simulink subsystem "encoder_8b10b"  (R2022b)
settings: Solver=VariableStepAuto  StartTime=0.0  StopTime=10.0  RelTol=1e-3
settings Model: Creator=Ali-Laptop  LastModifiedBy=Ali-Laptop

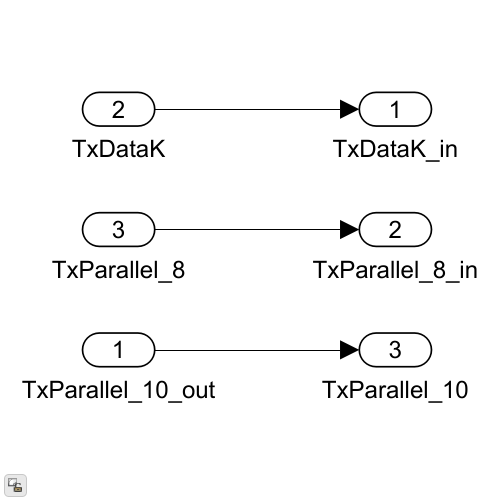
[thumbnail: Simulink's stored preview of the top-level diagram]
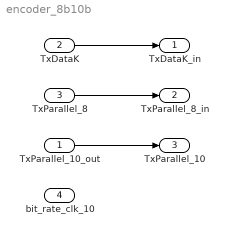
== system encoder_8b10b ==
  TxParallel_10_out : Inport
  TxDataK : Inport  Port=2
  TxParallel_8 : Inport  Port=3
  bit_rate_clk_10 : Inport  Port=4
  TxDataK_in : Outport
  TxParallel_8_in : Outport  Port=2
  TxParallel_10 : Outport  Port=3
  wires:
  TxParallel_10_out/1 -> TxParallel_10/1
  TxParallel_8/1 -> TxParallel_8_in/1
  TxDataK/1 -> TxDataK_in/1
